simulink model "Pendulo2GDL_RS"  (R2019b)
settings: Solver=VariableStepAuto  StartTime=0.0  StopTime=10.0  RelTol=1e-3
values from neighbouring files (symbols this model uses):
  C = [1 0 0 0]    [PenduloDatos.m]
  K = place(Al,Bl,[Pd1 Pd2 Pd3 Pd4])    [PenduloDatos.m]
  K0 = inv(C*(inv(-Al+Bl*K))*Bl)    [PenduloDatos.m]
  L = place(Al',C',[5*Pd1 5*Pd2 5*Pd3 5*Pd4])'    [PenduloDatos.m]
  Ref = 0.2    [PenduloDatos.m]
  XI = [0;0;0;0]    [PenduloDatos.m]
undefined symbols (not defined in the file or in its folder): Al, Bl
settings Model: Creator=ARQ SEVILLA R  LastModifiedBy=ARQ SEVILLA R

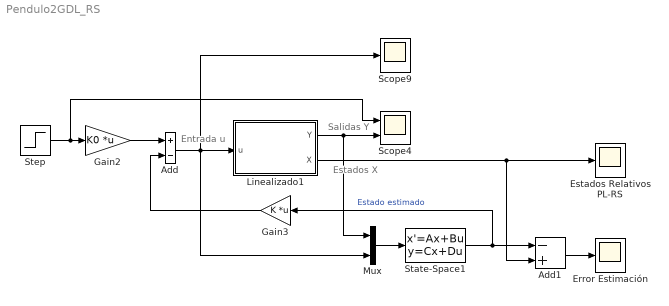
== system Pendulo2GDL_RS ==
  note: Entrada u
  note: Salidas Y
  note: Estados X
  Add : Sum  Inputs=+-
  Add1 : Sum  Inputs=-+
  Error Estimación : Scope
  Estados Relativos PL-RS : Scope
  Gain2 : Gain  Gain=K0  Multiplication=Matrix(K*u)
  Gain3 : Gain  Gain=K  Multiplication=Matrix(K*u)
  Linealizado1 : Subsystem
  Mux : Mux  Inputs=2
  Scope4 : Scope  NumInputPorts=2
  Scope9 : Scope
  State-Space1 : StateSpace  A=Al-L*C  B=[L,Bl]  C=eye(4)  D=zeros(4,2)  InitialCondition=XI
  Step : Step  Time=0  After=Ref  SampleTime=0
  wires:
  Step/1 -> Scope4/1, Gain2/1
  Add/1 -> Scope9/1, Linealizado1/1(u), Mux/2
  State-Space1/1 -> Add1/1, Gain3/1  "Estado estimado"
  Add1/1 -> Error Estimación/1
  Mux/1 -> State-Space1/1
  Gain2/1 -> Add/1
  Linealizado1/1(Y) -> Mux/1, Scope4/2
  Gain3/1 -> Add/2
  Linealizado1/2(X) -> Estados Relativos PL-RS/1, Add1/2

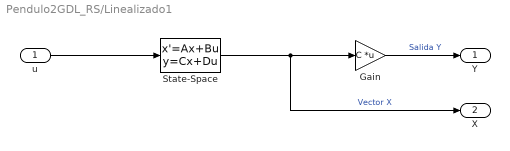
== system Pendulo2GDL_RS/Linealizado1 ==
  u : Inport
  Gain : Gain  Gain=C  Multiplication=Matrix(K*u)
  State-Space : StateSpace  A=Al  B=Bl  C=eye(4)  D=zeros(4,1)  InitialCondition=XI
  Y : Outport
  X : Outport  Port=2
  wires:
  u/1 -> State-Space/1
  Gain/1 -> Y/1  "Salida Y"
  State-Space/1 -> Gain/1, X/1  "Vector X"
